simulink model "ev_tms_v4"  (R2023a)
settings: Solver=VariableStepAuto  StartTime=0.0  StopTime=inf  RelTol=1e-3  AbsTol=1e-3
model workspace: external: MATLAB File /Users/rossschrader/Desktop/ML/ME/_Project/_v3/ev_tms_v3_params.m (data not in the file)
values from neighbouring files (symbols this model uses):
  ac_onoff = 0    [ev_tms_v4_params.m]
  battery_C1_LUT = [ ... (first row only)    [ev_tms_v4_params.m]
  battery_capacity_LUT = [28.0081 27.6250 27.6392]    [ev_tms_v4_params.m]
  battery_cell_cp = 795    [ev_tms_v4_params.m]
  battery_cell_mass = 2.5    [ev_tms_v4_params.m]
  battery_Em_LUT = [ ... (first row only)    [ev_tms_v4_params.m]
  battery_N_cells = 20    [ev_tms_v4_params.m]
  battery_Qe_init = 0    [ev_tms_v4_params.m]
  battery_R0_LUT = [ ... (first row only)    [ev_tms_v4_params.m]
  battery_R1_LUT = [ ... (first row only)    [ev_tms_v4_params.m]
  battery_SOC_LUT = [0 0.1 0.25 0.5 0.75 0.9 1]'    [ev_tms_v4_params.m]
  battery_T_init = init_T    (= 21)    [ev_tms_v4_params.m]
  battery_temperature_LUT = [5 20 40]    [ev_tms_v4_params.m]
  cabin_duct_area = 0.04    [ev_tms_v4_params.m]
  cabin_T_init = init_T    (= 21)    [ev_tms_v4_params.m]
  chiller_area_primary = chiller_N_tubes * pi * chiller_tube_D * chiller_tube_L    (= 0.439822971503)    [ev_tms_v4_params.m]
  chiller_N_baffles = 3    [ev_tms_v4_params.m]
  chiller_N_tubes = 100    [ev_tms_v4_params.m]
  chiller_tube_D = 0.0035    [ev_tms_v4_params.m]
  chiller_tube_L = 0.4    [ev_tms_v4_params.m]
  chiller_wall_conductivity = 240    [ev_tms_v4_params.m]
  chiller_wall_thickness = 1e-4    (= 0.0001)    [ev_tms_v4_params.m]
  compressor_rpm_LUT = [0, 1800, 3600]    [ev_tms_v4_params.m]
  condenser_air_area_flow = (condenser_N_tubes - 1) * condenser_L * condenser_gap_H    (= 0.3906)    [ev_tms_v4_params.m]
  condenser_air_area_primary = 2 * (condenser_N_tubes - 1) * condenser_W * (condenser_L + condenser_gap_H)    (= 1.4835)    [ev_tms_v4_params.m]
  condenser_W = 0.015    [ev_tms_v4_params.m]
  condenser_wall_conductivity = 240    [ev_tms_v4_params.m]
  condenser_wall_thickness = 1e-4    (= 0.0001)    [ev_tms_v4_params.m]
  coolant_channel_D = 0.0092    [ev_tms_v4_params.m]
  coolant_pipe_D = 0.019    [ev_tms_v4_params.m]
  coolant_T_init = init_T    (= 21)    [ev_tms_v4_params.m]
  coolant_tank_area = 0.11^2    (= 0.0121)    [ev_tms_v4_params.m]
  coolant_tank_volume = 5    [ev_tms_v4_params.m]
  coolant_valve_D_ratio_max = 0.95    [ev_tms_v4_params.m]
  coolant_valve_D_ratio_min = 1e-3    (= 0.001)    [ev_tms_v4_params.m]
  coolant_valve_displacement = 0.0063    [ev_tms_v4_params.m]
  coolant_valve_S_max = 0.0053    [ev_tms_v4_params.m]
  evaporator_air_area_flow = (evaporator_N_tubes - 1) * evaporator_L * evaporator_gap_H    (= 0.12)    [ev_tms_v4_params.m]
  evaporator_air_area_primary = 2 * (evaporator_N_tubes - 1) * evaporator_W * (evaporator_L + evaporator_gap_H)    (= 0.4323)    [ev_tms_v4_params.m]
  evaporator_P_target = 0.3    [ev_tms_v4_params.m]
  evaporator_W = 0.015    [ev_tms_v4_params.m]
  evaporator_wall_conductivity = 240    [ev_tms_v4_params.m]
  evaporator_wall_thickness = 1e-4    (= 0.0001)    [ev_tms_v4_params.m]
  pump_speed_max = 1000    [ev_tms_v4_params.m]
  radiator_air_area_flow = (radiator_N_tubes - 1) * radiator_L * radiator_gap_H    (= 0.0975)    [ev_tms_v4_params.m]
  radiator_air_area_primary = 2 * (radiator_N_tubes - 1) * radiator_W * (radiator_L + radiator_gap_H)    (= 0.436875)    [ev_tms_v4_params.m]
  radiator_W = 0.015    [ev_tms_v4_params.m]
  radiator_wall_conductivity = 240    [ev_tms_v4_params.m]
  radiator_wall_thickness = 1e-4    (= 0.0001)    [ev_tms_v4_params.m]
  refrigerant_alpha_init = 0.6    [ev_tms_v4_params.m]
  refrigerant_pipe_D = 0.01    [ev_tms_v4_params.m]
  T_env = t_(x)    [ev_tms_v4_params.m]
  T_setpoint = 20    [ev_tms_v4_params.m]
undefined symbols (not defined in the file or in its folder): bulb, outlet
libraries: fl_lib x221, nesl_utility x79, SimscapeFluids_lib x25, LiBatteryElements_lib x16, sdl_lib x3, slpidlib x2, simulink x1, rllib x1, autolibshared x1, SignalEditorBlockLib x1
(part 2 of 8)

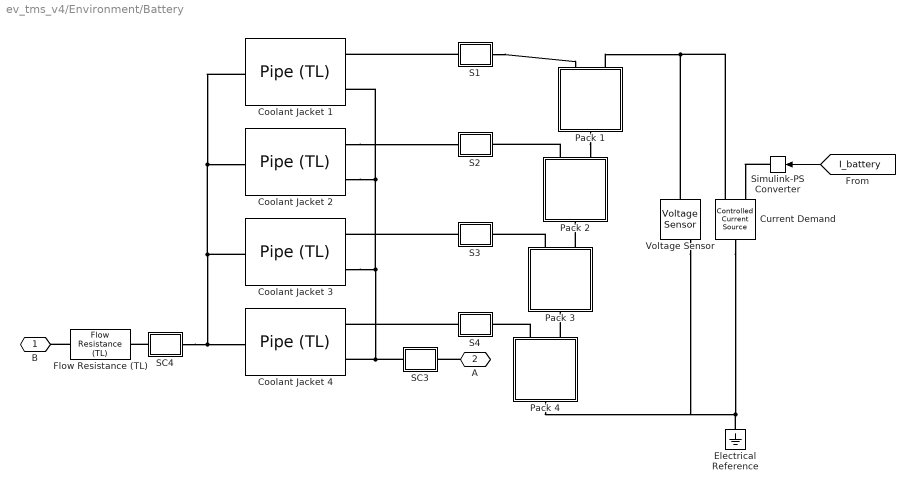
== system ev_tms_v4/Environment/Battery ==
  Coolant Jacket {1..4} (4 alike) : SimscapeFluids_lib/Thermal Liquid/Pipes & Fittings/Pipe (TL)  dynamic_compressibility=simscape.enum.onoff.on  inertia=simscape.enum.onoff.off  num_segments=1  pipe_length=0.7 m  cross_section_geometry=fluids.thermal_liquid.pipes_fittings.enum.CrossSectionGeometry.Custom  pipe_diameter=0.1 m  pipe_inner_diameter=0.05 m  pipe_outer_diameter=0.1 m  pipe_width=0.1 m  pipe_height=0.1 m  pipe_major_axis=0.1 m  pipe_minor_axis=0.05 m  pipe_side=0.1 m  pipe_angle=30 deg  area=pi * coolant_channel_D^2 / 4 m^2  Dh=coolant_channel_D m  wall_spec=fluids.thermal_liquid.pipes_fittings.enum.wall_spec.rigid  wall_compliance=1.2e-6 m/MPa  wall_time_constant=0.01 s  elevation_spec=foundation.enum.constant_variable.constant  elevation_gain=0 m  g=9.81 m/s^2  pressure_loss_spec=fluids.thermal_liquid.pipes_fittings.enum.PressureLossSpec.Haaland  local_pressure_loss_spec=fluids.thermal_liquid.pipes_fittings.enum.LocalLossSpec.AggregateLength  length_add=0 m  loss_coefficient=0.1  roughness_spec=fluids.thermal_liquid.pipes_fittings.enum.RoughnessSpec.Custom  roughness=1.5e-5 m  Re_friction_TLU=[ 400 1000 1.5e+3 3e+3 4e+3 6e+3 1e+4 2e+4 4e+4 6e+4 1e+5 1e+8 ]  friction_factor_TLU=[ 0.264 0.112 0.07099999999999999 0.0417 0.0387 0.0268 0.025 0.0232 0.0226 0.022 0.0214 0.0214 ]  shape_factor=64  Re_lam=100  Re_tur=500  mdot_nominal=[ 0.1 1 ] kg/s  p_diff_nominal=[ 0.001 0.01 ] MPa  mdot_threshold=1e-6 kg/s  heat_transfer_spec=fluids.thermal_liquid.pipes_fittings.enum.HeatTransferSpec.DittusBoelter  mdot_nominal_heat=[ 0.1 1 ] kg/s  T_in_nominal=[ 293.15 293.15 ] K  T_out_nominal=[ 300 300 ] K  p_in_nominal_heat=[ 0.101325 0.101325 ] MPa  T_wall_nominal=[ 303.15 303.15 ] K  a_coeff=0.3  b_Re_power=0.8  c_Pr_power=0.33  Nu_lam=3.66  Re_Colburn_TLU=[ 100 150 1000 ]  Colburn_factor_TLU=[ 0.019 0.013 0.002 ]  Re_Nu_TLU=[ 100 150 1000 ]  Pr_Nu_TLU=[ 1 10 ]  Nu_TLU=[ 3.72 4.21; 3.75 4.44; 4.21 7.15 ]  p0_vec=coolant_p_init MPa  T0_vec=coolant_T_init degC  mdot0=0.1 kg/s
  Current Demand : fl_lib/Electrical/Electrical Sources/Controlled Current Source
  Electrical Reference : fl_lib/Electrical/Electrical Elements/Electrical Reference
  Flow Resistance (TL) : fl_lib/Thermal Liquid/Elements/Flow Resistance (TL)  delta_p_nominal=1e-5 MPa  mdot_nominal=0.02 kg/s  area=pi * coolant_pipe_D^2 / 4 m^2  laminar_fraction=1e-3
  Pack 1 : Subsystem  Tag=PublishSubsystem  mask(Lithium cell (one RC-branch equivalent circuit)){Ncells=battery_N_cells, Qe_init=battery_Qe_init, T_init=battery_T_init + 273.15, Capacity_LUT=battery_capacity_LUT, Em_LUT=battery_Em_LUT, R0_LUT=battery_R0_LUT, R1_LUT=battery_R1_LUT, C1_LUT=battery_C1_LUT, cell_mass=battery_cell_mass, cell_Cp_heat=battery_cell_cp, SOC_LUT=battery_SOC_LUT, Temperature_LUT=battery_temperature_LUT + 273.15}
      mask prompts: Ncells "Number of series-connected cells"; Qe_init "Initial cell charge deficit (A*hr)"; T_init "Initial cell temperature (K)"; Capacity_LUT "Capacity (A*hr, 1xN table)"; Em_LUT "Em open-circuit voltage, Em (volts, MxN table)"; R0_LUT "R0 terminal resistance (ohms, MxN table)"; R1_LUT "R1 cell resistance (ohms, MxN table)"; C1_LUT "C1 capacitance (farads, MxN table)"; cell_mass "Cell mass (kg)"; cell_Cp_heat "Cell specific heat (J/kg/K)"; SOC_LUT "SOC table breakpoints (Mx1 array)"; Temperature_LUT "Temperature table breakpoints (K, 1xN array)"
      mask DialogControl ParameterTabVar0 Prompt: Main
      mask DialogControl ParameterTabVar01 Prompt: Electrical (per cell)
      mask DialogControl ParameterTabVar012 Prompt: Thermal (per cell)
      mask DialogControl ParameterTabVar0123 Prompt: Table Breakpoints
      mask Display:
      | % Battery icon
      | plot([2.8 1.3], [0 0])
      | plot([-0.2 -1.2 -1.2 -2.8], [0 0 -0.8 -0.8])
      | patch([1 1 -1 -1]*0.15 + 1.6, [-1 1 1 -1]*0.4, [0 0 0])
      | patch([1 1 -1 -1]*0.15 + 0.4, [-1 1 1 -1]*0.4, [0 0 0])
      | patch([1 1 -1 -1]*0.15 + 1.0, [-1 1 1 -1]*0.8, [0 0 0])
      | patch([1 1 -1 -1]*0.15 - 0.2, [-1 1 1 -1]*0.8, [0 0 0])
      | 
      | % Thermal port
      | plot([-1.4 -0.8], [1.2 1.2])
      | plot([-1.4 -0.8], [0.5 0.5])
      | plot([-1.4 -2.8], [0.8 0.8])
      | plot(0.2*sin(0:2*pi/50:2*pi) - 1.4, 0.35*cos(0:2*pi/50:2*pi) + 0.85)
      | plot(0.2*sin(0:2*pi/50:pi) - 0.8, 0.35*cos(0:2*pi/50:pi) + 0.85)
      | 
      | % Plot points to set plot range
      | color('white')
      | plot(2.8, 1.6)
      | plot(-2.8, -1.6)
      | 
      | % Port labels
      | color('red')
      | port_label('LConn', 1, 'H')
      | port_label('LConn', 2, '+')
      | port_label('RConn', 1, '-')
  Pack 2 : Subsystem  mask(Lithium cell (one RC-branch equivalent circuit)){Ncells=battery_N_cells, Qe_init=battery_Qe_init, T_init=battery_T_init + 273.15, Capacity_LUT=battery_capacity_LUT, Em_LUT=battery_Em_LUT, R0_LUT=battery_R0_LUT, R1_LUT=battery_R1_LUT, C1_LUT=battery_C1_LUT, cell_mass=battery_cell_mass, cell_Cp_heat=battery_cell_cp, SOC_LUT=battery_SOC_LUT, Temperature_LUT=battery_temperature_LUT + 273.15}
      mask prompts: Ncells "Number of series-connected cells"; Qe_init "Initial cell charge deficit (A*hr)"; T_init "Initial cell temperature (K)"; Capacity_LUT "Capacity (A*hr, 1xN table)"; Em_LUT "Em open-circuit voltage, Em (volts, MxN table)"; R0_LUT "R0 terminal resistance (ohms, MxN table)"; R1_LUT "R1 cell resistance (ohms, MxN table)"; C1_LUT "C1 capacitance (farads, MxN table)"; cell_mass "Cell mass (kg)"; cell_Cp_heat "Cell specific heat (J/kg/K)"; SOC_LUT "SOC table breakpoints (Mx1 array)"; Temperature_LUT "Temperature table breakpoints (K, 1xN array)"
      mask DialogControl ParameterTabVar0 Prompt: Main
      mask DialogControl ParameterTabVar01 Prompt: Electrical (per cell)
      mask DialogControl ParameterTabVar012 Prompt: Thermal (per cell)
      mask DialogControl ParameterTabVar0123 Prompt: Table Breakpoints
      mask Display:
      | % Battery icon
      | plot([2.8 1.3], [0 0])
      | plot([-0.2 -1.2 -1.2 -2.8], [0 0 -0.8 -0.8])
      | patch([1 1 -1 -1]*0.15 + 1.6, [-1 1 1 -1]*0.4, [0 0 0])
      | patch([1 1 -1 -1]*0.15 + 0.4, [-1 1 1 -1]*0.4, [0 0 0])
      | patch([1 1 -1 -1]*0.15 + 1.0, [-1 1 1 -1]*0.8, [0 0 0])
      | patch([1 1 -1 -1]*0.15 - 0.2, [-1 1 1 -1]*0.8, [0 0 0])
      | 
      | % Thermal port
      | plot([-1.4 -0.8], [1.2 1.2])
      | plot([-1.4 -0.8], [0.5 0.5])
      | plot([-1.4 -2.8], [0.8 0.8])
      | plot(0.2*sin(0:2*pi/50:2*pi) - 1.4, 0.35*cos(0:2*pi/50:2*pi) + 0.85)
      | plot(0.2*sin(0:2*pi/50:pi) - 0.8, 0.35*cos(0:2*pi/50:pi) + 0.85)
      | 
      | % Plot points to set plot range
      | color('white')
      | plot(2.8, 1.6)
      | plot(-2.8, -1.6)
      | 
      | % Port labels
      | color('red')
      | port_label('LConn', 1, 'H')
      | port_label('LConn', 2, '+')
      | port_label('RConn', 1, '-')
  Pack 3 : Subsystem  mask(Lithium cell (one RC-branch equivalent circuit)){Ncells=battery_N_cells, Qe_init=battery_Qe_init, T_init=battery_T_init + 273.15, Capacity_LUT=battery_capacity_LUT, Em_LUT=battery_Em_LUT, R0_LUT=battery_R0_LUT, R1_LUT=battery_R1_LUT, C1_LUT=battery_C1_LUT, cell_mass=battery_cell_mass, cell_Cp_heat=battery_cell_cp, SOC_LUT=battery_SOC_LUT, Temperature_LUT=battery_temperature_LUT + 273.15}
      mask prompts: Ncells "Number of series-connected cells"; Qe_init "Initial cell charge deficit (A*hr)"; T_init "Initial cell temperature (K)"; Capacity_LUT "Capacity (A*hr, 1xN table)"; Em_LUT "Em open-circuit voltage, Em (volts, MxN table)"; R0_LUT "R0 terminal resistance (ohms, MxN table)"; R1_LUT "R1 cell resistance (ohms, MxN table)"; C1_LUT "C1 capacitance (farads, MxN table)"; cell_mass "Cell mass (kg)"; cell_Cp_heat "Cell specific heat (J/kg/K)"; SOC_LUT "SOC table breakpoints (Mx1 array)"; Temperature_LUT "Temperature table breakpoints (K, 1xN array)"
      mask DialogControl ParameterTabVar0 Prompt: Main
      mask DialogControl ParameterTabVar01 Prompt: Electrical (per cell)
      mask DialogControl ParameterTabVar012 Prompt: Thermal (per cell)
      mask DialogControl ParameterTabVar0123 Prompt: Table Breakpoints
      mask Display:
      | % Battery icon
      | plot([2.8 1.3], [0 0])
      | plot([-0.2 -1.2 -1.2 -2.8], [0 0 -0.8 -0.8])
      | patch([1 1 -1 -1]*0.15 + 1.6, [-1 1 1 -1]*0.4, [0 0 0])
      | patch([1 1 -1 -1]*0.15 + 0.4, [-1 1 1 -1]*0.4, [0 0 0])
      | patch([1 1 -1 -1]*0.15 + 1.0, [-1 1 1 -1]*0.8, [0 0 0])
      | patch([1 1 -1 -1]*0.15 - 0.2, [-1 1 1 -1]*0.8, [0 0 0])
      | 
      | % Thermal port
      | plot([-1.4 -0.8], [1.2 1.2])
      | plot([-1.4 -0.8], [0.5 0.5])
      | plot([-1.4 -2.8], [0.8 0.8])
      | plot(0.2*sin(0:2*pi/50:2*pi) - 1.4, 0.35*cos(0:2*pi/50:2*pi) + 0.85)
      | plot(0.2*sin(0:2*pi/50:pi) - 0.8, 0.35*cos(0:2*pi/50:pi) + 0.85)
      | 
      | % Plot points to set plot range
      | color('white')
      | plot(2.8, 1.6)
      | plot(-2.8, -1.6)
      | 
      | % Port labels
      | color('red')
      | port_label('LConn', 1, 'H')
      | port_label('LConn', 2, '+')
      | port_label('RConn', 1, '-')
  Pack 4 : Subsystem  mask(Lithium cell (one RC-branch equivalent circuit)){Ncells=battery_N_cells, Qe_init=battery_Qe_init, T_init=battery_T_init + 273.15, Capacity_LUT=battery_capacity_LUT, Em_LUT=battery_Em_LUT, R0_LUT=battery_R0_LUT, R1_LUT=battery_R1_LUT, C1_LUT=battery_C1_LUT, cell_mass=battery_cell_mass, cell_Cp_heat=battery_cell_cp, SOC_LUT=battery_SOC_LUT, Temperature_LUT=battery_temperature_LUT + 273.15}
      mask prompts: Ncells "Number of series-connected cells"; Qe_init "Initial cell charge deficit (A*hr)"; T_init "Initial cell temperature (K)"; Capacity_LUT "Capacity (A*hr, 1xN table)"; Em_LUT "Em open-circuit voltage, Em (volts, MxN table)"; R0_LUT "R0 terminal resistance (ohms, MxN table)"; R1_LUT "R1 cell resistance (ohms, MxN table)"; C1_LUT "C1 capacitance (farads, MxN table)"; cell_mass "Cell mass (kg)"; cell_Cp_heat "Cell specific heat (J/kg/K)"; SOC_LUT "SOC table breakpoints (Mx1 array)"; Temperature_LUT "Temperature table breakpoints (K, 1xN array)"
      mask DialogControl ParameterTabVar0 Prompt: Main
      mask DialogControl ParameterTabVar01 Prompt: Electrical (per cell)
      mask DialogControl ParameterTabVar012 Prompt: Thermal (per cell)
      mask DialogControl ParameterTabVar0123 Prompt: Table Breakpoints
      mask Display:
      | % Battery icon
      | plot([2.8 1.3], [0 0])
      | plot([-0.2 -1.2 -1.2 -2.8], [0 0 -0.8 -0.8])
      | patch([1 1 -1 -1]*0.15 + 1.6, [-1 1 1 -1]*0.4, [0 0 0])
      | patch([1 1 -1 -1]*0.15 + 0.4, [-1 1 1 -1]*0.4, [0 0 0])
      | patch([1 1 -1 -1]*0.15 + 1.0, [-1 1 1 -1]*0.8, [0 0 0])
      | patch([1 1 -1 -1]*0.15 - 0.2, [-1 1 1 -1]*0.8, [0 0 0])
      | 
      | % Thermal port
      | plot([-1.4 -0.8], [1.2 1.2])
      | plot([-1.4 -0.8], [0.5 0.5])
      | plot([-1.4 -2.8], [0.8 0.8])
      | plot(0.2*sin(0:2*pi/50:2*pi) - 1.4, 0.35*cos(0:2*pi/50:2*pi) + 0.85)
      | plot(0.2*sin(0:2*pi/50:pi) - 0.8, 0.35*cos(0:2*pi/50:pi) + 0.85)
      | 
      | % Plot points to set plot range
      | color('white')
      | plot(2.8, 1.6)
      | plot(-2.8, -1.6)
      | 
      | % Port labels
      | color('red')
      | port_label('LConn', 1, 'H')
      | port_label('LConn', 2, '+')
      | port_label('RConn', 1, '-')
  S1 : Subsystem
      mask Display: disp(get_param(gcb, 'Name'))
  S2 : Subsystem
      mask Display: disp(get_param(gcb, 'Name'))
  S3 : Subsystem
      mask Display: disp(get_param(gcb, 'Name'))
  S4 : Subsystem
      mask Display: disp(get_param(gcb, 'Name'))
  SC3 : Subsystem
      mask Display: disp(get_param(gcb, 'Name'))
  SC4 : Subsystem
      mask Display: disp(get_param(gcb, 'Name'))
  Simulink-PS Converter : nesl_utility/Simulink-PS Converter  PhysicalDomain=network_engine_domain  SubClassName=ps_input  LeftPortType=input  RightPortType=output  PseudoPeriodic=off  Frequencies=[]  NoiseDistribution=none  NoiseParameters=[]  Unit=A  AffineConversion=off  FilteringAndDerivatives=provide  SimscapeFilterOrder=1  InputFilterTimeConstant=0.001  UdotUserProvided=0
  Voltage Sensor : fl_lib/Electrical/Electrical Sensors/Voltage Sensor
  B : PMIOPort  Side=Left
  A : PMIOPort  Port=2  Side=Right
  wires:
  [I_battery] -> Simulink-PS Converter/1
  connections:
  Current Demand/LConn1 -- Pack 4/RConn1 -- Voltage Sensor/RConn2 -- Electrical Reference/LConn1
  Current Demand/RConn2 -- Pack 1/LConn2 -- Voltage Sensor/LConn1
  Simulink-PS Converter/RConn1 -- Current Demand/RConn1
  S1/LConn1 -- Coolant Jacket 1/LConn2
  S3/LConn1 -- Coolant Jacket 3/LConn2
  S4/LConn1 -- Coolant Jacket 4/LConn2
  Pack 1/RConn1 -- Pack 2/LConn2
  Pack 3/LConn2 -- Pack 2/RConn1
  Pack 4/LConn2 -- Pack 3/RConn1
  Pack 2/LConn1 -- S2/RConn1
  Coolant Jacket 3/LConn1 -- SC3/LConn1 -- Coolant Jacket 4/LConn1 -- Coolant Jacket 1/LConn1 -- Coolant Jacket 2/LConn1
  S1/RConn1 -- Pack 1/LConn1
  Coolant Jacket 2/LConn2 -- S2/LConn1
  Pack 3/LConn1 -- S3/RConn1
  Pack 4/LConn1 -- S4/RConn1
  A/RConn1 -- SC3/RConn1
  Coolant Jacket 3/RConn1 -- Coolant Jacket 2/RConn1 -- Coolant Jacket 1/RConn1 -- SC4/RConn1 -- Coolant Jacket 4/RConn1
  SC4/LConn1 -- Flow Resistance (TL)/LConn1
  Flow Resistance (TL)/RConn1 -- B/RConn1

== system ev_tms_v4/Environment/Battery Pump ==
  Battery Pump : SimscapeFluids_lib/Thermal Liquid/Pumps & Motors/Fixed-Displacement Pump (TL)  loss_spec=1  displacement=pump_displacement l/rev  omega_nominal=0.5 * pump_speed_max rpm  p_nominal=0.1 MPa  mu_nominal=0.9 cP  vol_eff_nominal=0.92  mech_eff_nominal=0.88  no_load_torque=0.03 N*m  p_diff_eff_TLU=[.1, 1, 2] MPa  omega_eff_TLU=[25, 50, 100, 200, 300, 400] rad/s  vol_eff_TLU=[.816, .908, .954, .977, .981, .984; .325, .663, .831, .916, .925, .946; .137, .568, .78, .892, .893, .91]  mech_eff_TLU=[.996, .996, .996, .996, .996, .996; .988, .989, .989, .989, .989, .99; .981, .981, .982, .982, .983, .984]  p_diff_loss_TLU=[.1, 1, 2] MPa  omega_loss_TLU=[25, 50, 100, 200, 300, 400] rad/s  vol_loss_TLU=[.023, .023, .023, .023, .0285, .032; .0844, .0842, .0845, .084, .1125, .108; .1079, .108, .11, .108, .1605, .18] * 1e-3 m^3/s  mech_loss_TLU=[.002, .002, .002, .002, .002, .002; .0607, .0556, .0556, .0556, .0556, .0505; .1937, .1937, .1833, .1833, .1729, .1626] N*m  vol_eff_min=1e-3  vol_eff_max=1  mech_eff_min=1e-3  mech_eff_max=1  pressure_threshold=1e-3 MPa  omega_threshold=10 rad/s  area=pi * coolant_pipe_D^2 / 4 m^2  quadrant_check=0  pump_mode_check=simscape.enum.assert.action.none
  From1 : From  Commented=on  GotoTag=cmd_battery_pump_2
  Ideal Angular Velocity Source : fl_lib/Mechanical/Mechanical Sources/Ideal Angular Velocity Source
  Max Speed [rpm] : Gain  Gain=pump_speed_max
  Mechanical Rotational Reference : fl_lib/Mechanical/Rotational Elements/Mechanical Rotational Reference
  PS-Simulink Converter : nesl_utility/PS-Simulink Converter  PhysicalDomain=network_engine_domain  SubClassName=ps_output  LeftPortType=input  RightPortType=output  PseudoPeriodic=off  Frequencies=[]  VectorFormat=inherit  Unit=inherit  AffineConversion=off
  Rotational Power Sensor : sdl_lib/Sensors/Rotational Power Sensor  measurement_type=sdl.enum.rotationalPowerSensorType.instantaneous  averaging_period=1 s  max_frequency=1000 Hz  max_speed=1000 rpm
      settings: InternalSimscapePortConfiguration="{\"Bottom\":[],\"Left\":[{\"id\":\"S\",\"label\":\"S\",\"type\":\"foundation.mechanical.rotational.rotational\"},{\"id\":\"R\",\"label\":\"R\",\"type\":\"foundation.mechanical.rotational.rotational\"},{\"id\":\"C\",\"label\":\"C\",\"type\":\"foundation.mechanical.rotational.rotational\"}],\"Right\":[{\"id\":\"P\",\"label\":\"P\",\"type\":\"output\"}],\"Top\":[]}"
  Simulink-PS Converter : nesl_utility/Simulink-PS Converter  PhysicalDomain=network_engine_domain  SubClassName=ps_input  LeftPortType=input  RightPortType=output  PseudoPeriodic=off  Frequencies=[]  NoiseDistribution=none  NoiseParameters=[]  Unit=rpm  AffineConversion=off  FilteringAndDerivatives=provide  SimscapeFilterOrder=1  InputFilterTimeConstant=0.001  UdotUserProvided=0
  Transfer Fcn : TransferFcn  Denominator=[5 1]
  A : PMIOPort  Side=Left
  B : PMIOPort  Port=2  Side=Right
  tag scope: bat_pump_pwr=global
  wires:
  Max Speed [rpm]/1 -> Simulink-PS Converter/1
  Transfer Fcn/1 -> Max Speed [rpm]/1
  PS-Simulink Converter/1 -> [bat_pump_pwr]
  [cmd_battery_pump] -> Transfer Fcn/1
  connections:
  Battery Pump/LConn2 -- B/RConn1
  Battery Pump/LConn1 -- A/RConn1
  Battery Pump/RConn2 -- Rotational Power Sensor/LConn3 -- Mechanical Rotational Reference/LConn1 -- Ideal Angular Velocity Source/RConn2
  Simulink-PS Converter/RConn1 -- Ideal Angular Velocity Source/RConn1
  Ideal Angular Velocity Source/LConn1 -- Rotational Power Sensor/LConn1
  Battery Pump/RConn1 -- Rotational Power Sensor/LConn2
  PS-Simulink Converter/LConn1 -- Rotational Power Sensor/RConn1

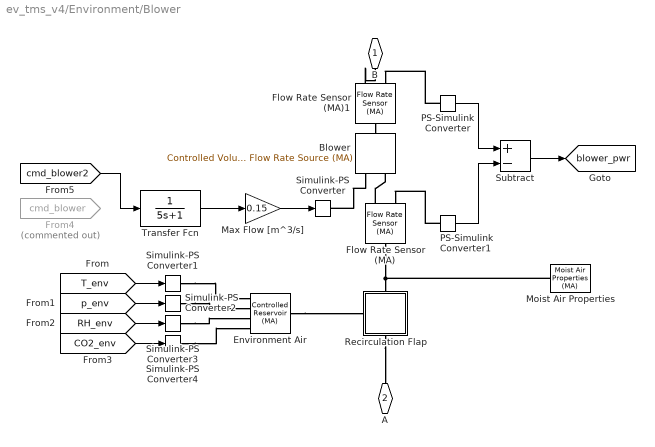
== system ev_tms_v4/Environment/Blower ==
  Blower : fl_lib/Moist Air/Sources/Controlled Volumetric Flow Rate Source (MA)  power_spec=foundation.enum.power_spec.isentropic  volumetric_flow_conditions=foundation.enum.volumetric_flow_conditions.actual  p_std=0.101325 MPa  T_std=20 degC  RH_std=0.65  area_A=cabin_duct_area m^2  area_B=cabin_duct_area m^2
      settings: InternalSimscapePortConfiguration="{\"Bottom\":[],\"Left\":[{\"id\":\"A\",\"label\":\"A\",\"type\":\"foundation.moist_air.moist_air\"},{\"id\":\"V\",\"label\":\"V\",\"type\":\"input\"}],\"Right\":[{\"id\":\"B\",\"label\":\"B\",\"type\":\"foundation.moist_air.moist_air\"}],\"Top\":[]}"
  Environment Air : fl_lib/Moist Air/Elements/Controlled Reservoir (MA)  moisture_spec=foundation.enum.moisture_spec.relative_humidity  trace_gas_spec=foundation.enum.trace_gas_spec.mole_fraction  RH_ws=1  area_A=cabin_duct_area m^2  input_error_spec=foundation.enum.input_range_error.warn
      settings: InternalSimscapePortConfiguration="{\"Bottom\":[],\"Left\":[{\"id\":\"A\",\"label\":\"A\",\"type\":\"foundation.moist_air.moist_air\"}],\"Right\":[{\"id\":\"T\",\"label\":\"T\",\"type\":\"input\"},{\"id\":\"P\",\"label\":\"P\",\"type\":\"input\"},{\"id\":\"W\",\"label\":\"W\",\"type\":\"input\"},{\"id\":\"G\",\"label\":\"G\",\"type\":\"input\"}],\"Top\":[]}"
  Flow Rate Sensor (MA) : fl_lib/Moist Air/Sensors/Flow Rate Sensor (MA)  mass_flow_measure=false  volumetric_flow_measure=false  volumetric_flow_conditions=foundation.enum.volumetric_flow_conditions.actual  p_std=0.101325 MPa  T_std=20 degC  RH_std=0.65  energy_flow_measure=true  vapor_flow_measure=false  gas_flow_measure=false
      settings: InternalSimscapePortConfiguration="{\"Bottom\":[{\"id\":\"PHI\",\"label\":\"φ\",\"type\":\"output\"}],\"Left\":[{\"id\":\"A\",\"label\":\"A\",\"type\":\"foundation.moist_air.moist_air\"}],\"Right\":[{\"id\":\"B\",\"label\":\"B\",\"type\":\"foundation.moist_air.moist_air\"}],\"Top\":[]}"
  Flow Rate Sensor (MA)1 : fl_lib/Moist Air/Sensors/Flow Rate Sensor (MA)  mass_flow_measure=false  volumetric_flow_measure=false  volumetric_flow_conditions=foundation.enum.volumetric_flow_conditions.actual  p_std=0.101325 MPa  T_std=20 degC  RH_std=0.65  energy_flow_measure=true  vapor_flow_measure=false  gas_flow_measure=false
      settings: InternalSimscapePortConfiguration="{\"Bottom\":[{\"id\":\"PHI\",\"label\":\"φ\",\"type\":\"output\"}],\"Left\":[{\"id\":\"A\",\"label\":\"A\",\"type\":\"foundation.moist_air.moist_air\"}],\"Right\":[{\"id\":\"B\",\"label\":\"B\",\"type\":\"foundation.moist_air.moist_air\"}],\"Top\":[]}"
  From4 : From  Commented=on  GotoTag=cmd_blower  TagVisibility=global
  Max Flow [m^3/s] : Gain  Gain=0.15
  Moist Air Properties : fl_lib/Moist Air/Utilities/Moist Air Properties (MA)  R_a=287.047 J/kg/K  T_TLU=[-56.55, -50 : 10 : -10, -5 : 1 : 5, 10 : 10 : 350]' degC  h_a_TLU=[342.416126230579; 349.005511058471; 359.063577249119; 369.119948684177; 379.175469465129; 389.230944678417; 394.258910928084; 395.264534937366; 396.27017101329; 397.275819932805; 398.281482472874; 399.287159410541; 400.292851523015; 401.298559587728; 402.304284382408; 403.310026685143; 404.315787274435; 409.34489180313; 419.404921755863; 429.468036401264; 439.535033154839; 449.606720928652; 459.683919949603; 469.767460521911; 479.858181001348; 489.956925196484; 500.064539372946; 510.181869006204; 520.309755403634; 530.449032296018; 540.60052248087; 550.765034584465; 560.943359995745; 571.136270013102; 581.344513234296; 591.568813210327; 601.809866375885; 612.068340261954; 622.344871990218; 632.640067043998; 642.95449830646; 653.288705353699; 663.643193987949; 674.018435994423; 684.414869104228; 694.832897145098; 705.272890361557; 715.735185886199; 726.220088344236; 736.727870574087; 747.258774447567; 757.813011774199] kJ/kg  mu_a_TLU=[14.2568883320012; 14.6140127728333; 15.1517277055779; 15.6806860159119; 16.2012351072083; 16.7137043125028; 16.9670071730589; 17.017438062815; 17.0677930842452; 17.1180725309876; 17.1682766951315; 17.2184058672268; 17.2684603362935; 17.3184403898301; 17.3683463138234; 17.4181783927569; 17.4679369096204; 17.7156358640698; 18.2056751785154; 18.68879035749; 19.1652344664982; 19.6352478927873; 20.099059103658; 20.5568853601578; 21.0089333871663; 21.4554000014051; 21.8964726992323; 22.3323302062775; 22.7631429910631; 23.1890737447833; 23.6102778293792; 24.0269036959922; 24.4390932757886; 24.8469823450548; 25.2507008663546; 25.6503733074314; 26.0461189394339; 26.4380521159325; 26.8262825340948; 27.2109154792923; 27.5920520543128; 27.969789394274; 28.3442208682439; 28.7154362685068; 29.0835219883356; 29.4485611890712; 29.8106339572472; 30.1698174524429; 30.5261860464955; 30.8798114546565; 31.2307628592324; 31.5791070262086] s*uPa  k_a_TLU=[19.8808489374933; 20.4162454629695; 21.2248743590758; 22.0232452890903; 22.8117314495857; 23.5906913619588; 23.9767075412237; 24.053639990175; 24.1304826682191; 24.2072359051629; 24.2839000294007; 24.3604753679152; 24.4369622462801; 24.5133609886625; 24.5896719178249; 24.6658953551279; 24.7420316205333; 25.1214164701832; 25.8738283029331; 26.6180150229276; 27.3542674377332; 28.0828634735341; 28.8040686837224; 29.5181367785657; 30.2253101618423; 30.9258204644224; 31.6198890677835; 32.3077276126633; 32.9895384896798; 33.6655153099498; 34.33584335461; 35.0007000027879; 35.6602551380254; 36.3146715334901; 36.9641052165342; 37.6087058133173; 38.248616874307; 38.8839761815308; 39.5149160384798; 40.1415635435708; 40.7640408480637; 41.3824653993118; 41.9969501701893; 42.6076038755117; 43.2145311762238; 43.8178328720941; 44.4176060836121; 45.013944423749; 45.6069381602018; 46.1966743687041; 46.783237077953; 47.3667074066625] mW/m/K  p_min=1 kPa  p_max=inf MPa  T_min=-56.55 degC  T_max=350 degC  properties_range_check=simscape.enum.assert.action.error  p_atm=0.101325 MPa  T_atm=20 degC  R_w=461.523 J/kg/K  p_ws_TLU=[1.71168953425982e-06; 3.93770601979424e-06; 1.28411717710344e-05; 3.80051394873809e-05; .00010323902900209; .000259873810798063; .000401741022116384; .000437454836117844; .000476040820618202; .000517704666185737; .000562664883741207; .000611212677444345; .000657088049117899; .000705987905898279; .000758082381149132; .000813549384183233; .000872574861129522; .00122818386934022; .0023392147667769; .00424668834054807; .00738442748706953; .0123512704340234; .0199458019246787; .0312006356960619; .0474147199263783; .0701823607447713; .10141797792131; .143375967241115; .198665399739302; .270259606559999; .361500961984849; .476101381081492; .618139196722055; .792053183687694; 1.0026345688121; 1.25501792086105; 1.55467186826983; 1.90739066433297; 2.31928772772542; 2.79679245576864; 3.34665187151016; 3.97593907083533; 4.69207105435535; 5.5028394740883; 6.41645928168037; 7.4416425436169; 8.58770832955728; 9.86474556030261; 11.2838558865497; 12.8575218898034; 14.6001810568052; 16.5291642526045] MPa  h_w_vap_TLU=[2836.88241275372; 2837.81392500514; 2838.63937175807; 2838.7309929628; 2838.06905313927; 2836.62597341095; 2835.60023952573; 2835.37006381376; 2835.13143158077; 2834.88429145066; 2834.62859062897; 2500.93420564316; 2498.55329907119; 2496.17495082036; 2493.79885912205; 2491.42474723191; 2489.05236104642; 2477.20875029194; 2453.54955988604; 2429.83856603313; 2406.00136954922; 2381.97406342174; 2357.69101156389; 2333.08088387814; 2308.06565480412; 2282.56034405021; 2256.47287422313; 2229.70428017508; 2202.14968030993; 2173.69998896199; 2144.24368406447; 2113.66758247452; 2081.85585110571; 2048.68725710494; 2014.03141249899; 1977.7449923284; 1939.66849592886; 1899.62342931686; 1857.40930169838; 1812.79975416601; 1765.53721731251; 1715.32525772152; 1661.81700477787; 1604.59703745016; 1543.1534616334; 1476.83692476464; 1404.80240352424; 1325.92091736114; 1238.61667822208; 1140.5102987018; 1027.62017777647; 892.733785613825] kJ/kg  h_w_TLU=[2396.55944251649; 2408.68643343608; 2427.1988031141; 2445.702165897; 2464.18429108356; 2482.62529466839; 2491.82135326629; 2493.6580151792; 2495.49372578218; 2497.32843835745; 2499.16210446923; 2500.99462758899; 2502.83092214066; 2504.6665223621; 2506.50140563013; 2508.335548891; 2510.16892865793; 2519.32352241995; 2537.56068088674; 2555.67742615292; 2573.6403223998; 2591.4109179101; 2608.9455037701; 2626.19492016262; 2643.10444358428; 2659.61377634497; 2675.58278696023; 2696.1846256545; 2716.49989553741; 2736.6235210957; 2756.61216047011; 2776.50561773853; 2796.33378922508; 2816.11979583049; 2835.88181423877; 2855.63430574511; 2875.38889327595; 2895.15500577172; 2914.94035964689; 2934.75132290228; 2954.59319330244; 2974.47041285505; 2994.38673458964; 3014.34535328009; 3034.34900867103; 3054.40006755764; 3074.50058946898; 3094.65237953784; 3114.85703128106; 3135.11596137801; 3155.43043805905; 3175.80160435813] kJ/kg  mu_w_TLU=[6.81365662228272; 7.04953750742707; 7.40970098298307; 7.76991278093907; 8.13017290129507; 8.49048134405107; 8.67065368632907; 8.70668960445667; 8.74272600580827; 8.77876289038387; 8.81480025818347; 8.85083810920707; 8.88687644345467; 8.92291526092627; 8.95895456162187; 8.99499434554147; 9.03103461268507; 9.21124319676307; 9.57169660671907; 9.93219833907507; 10.2927483938311; 10.6533467709871; 11.0139934705431; 11.3746884924991; 11.7354318368551; 12.0962235036111; 12.4570634927671; 12.8179518043231; 13.1788884382791; 13.5398733946351; 13.9009066733911; 14.2619882745471; 14.6231181981031; 14.9842964440591; 15.3455230124151; 15.7067979031711; 16.0681211163271; 16.4294926518831; 16.7909125098391; 17.1523806901951; 17.5138971929511; 17.8754620181071; 18.2370751656631; 18.5987366356191; 18.9604464279751; 19.3222045427311; 19.6840109798871; 20.0458657394431; 20.4077688213991; 20.7697202257551; 21.1317199525111; 21.4937680016671] s*uPa  k_w_TLU=[11.46288215976; 11.941997488935; 12.676358586935; 13.414208884935; 14.155548382935; 14.900377080935; 15.274099879935; 15.348949115735; 15.423833243535; 15.498752263335; 15.573706175135; 15.648694978935; 15.723718674735; 15.798777262535; 15.873870742335; 15.948999114135; 16.024162377935; 16.400502076935; 17.155798374935; 17.914583872935; 18.676858570935; 19.442622468935; 20.211875566935; 20.984617864935; 21.760849362935; 22.540570060935; 23.323779958935; 24.110479056935; 24.900667354935; 25.694344852935; 26.491511550935; 27.292167448935; 28.096312546935; 28.903946844935; 29.715070342935; 30.529683040935; 31.347784938935; 32.169376036935; 32.994456334935; 33.823025832935; 34.655084530935; 35.490632428935; 36.329669526935; 37.172195824935; 38.018211322935; 38.867716020935; 39.720709918935; 40.577193016935; 41.437165314935; 42.300626812935; 43.167577510935; 44.038017408935] mW/m/K  D_w=25 mm^2/s  trace_gas_model=foundation.enum.trace_gas_model.track_fraction  R_g=188.923 J/kg/K  h_g_TLU=[439.555216260064; 444.670268200251; 452.538618847003; 460.487124258496; 468.522588768941; 476.649415958793; 480.74798538725; 481.57054318762; 482.394052398751; 483.218514288831; 484.043930029015; 484.870300696555; 485.697627277859; 486.525910671489; 487.355151691079; 488.185351068185; 489.016509455051; 493.186704139431; 501.599194953048; 510.107689961685; 518.711611080182; 527.410026793075; 536.201764778798; 545.085474203452; 554.059675505208; 563.122805485367; 572.27325096919; 581.509373027928; 590.829525105886; 600.232066705818; 609.715373581392; 619.277845178105; 628.917909922924; 638.634028838794; 648.424697859328; 658.288449140109; 668.223851601449; 678.229510889093; 688.304068901113; 698.44620299875; 708.654624994591; 718.928079991818; 729.265345132425; 739.665228299475; 750.126566808087; 760.648226111439; 771.229098541268; 781.868102096908; 792.564179292476; 803.316296068366; 814.123440770426; 824.984623198037] kJ/kg  mu_g_TLU=[10.8921054191698; 11.2215357085649; 11.7233300740382; 12.2234238147811; 12.7215124453467; 13.2173328890673; 13.4643203184773; 13.5136406274989; 13.562934752385; 13.6122025024997; 13.6614436900741; 13.7106581301692; 13.7598456406398; 13.8090060420983; 13.8581391578796; 13.9072448140062; 13.9563228391538; 14.2012926853717; 14.6890687376044; 15.1738428124161; 15.6554929043332; 16.1339159800463; 16.6090257998657; 17.0807510097148; 17.5490334645512; 18.0138267508952; 18.4750948814453; 18.9328111390399; 19.3869570507278; 19.8375214755778; 20.2844997922255; 20.7278931741254; 21.1677079421287; 21.6039549853963; 22.036649242835; 22.4658092382469; 22.8914566632375; 23.3136160026627; 23.7323141980278; 24.1475803447965; 24.5594454200432; 24.9679420372927; 25.3731042257492; 25.774967231431; 26.1735673380029; 26.5689417053362; 26.9611282240413; 27.350165384404; 27.73609215832; 28.118947892972; 28.4987722151178; 28.8756049449796] s*uPa  k_g_TLU=[10.489430678843; 10.9507672150864; 11.666197960308; 12.392559739764; 13.1299519771612; 13.8778409888416; 14.2554325416312; 14.3312274189707; 14.4071122346908; 14.4830860227061; 14.5591478179508; 14.6352966574703; 14.7115315815553; 14.787851634907; 14.8642558678259; 14.9407433374142; 15.0173131087819; 15.401364480906; 16.1751373988038; 16.9558134611595; 17.7432208682398; 18.5366976599676; 19.3360988502003; 20.1412225692689; 20.9517507672929; 21.7672310558863; 22.5871115634685; 23.4107980865695; 24.2377021890869; 25.0672663781241; 25.8989689893876; 26.732318357514; 27.5668446164644; 28.4020933015927; 29.2376215872816; 30.0729965057542; 30.9077942826816; 31.7416001931033; 32.5740086297993; 33.4046232539953; 34.2330571812868; 35.0589331874899; 35.8818839295189; 36.701552179391; 37.5175910702657; 38.3296643536716; 39.1374466671854; 39.9406238119064; 40.7388930391313; 41.5319633456945; 42.3195557774861; 43.1014037407076] mW/m/K  D_g=16 mm^2/s
  PS-Simulink Converter : nesl_utility/PS-Simulink Converter  PhysicalDomain=network_engine_domain  SubClassName=ps_output  LeftPortType=input  RightPortType=output  PseudoPeriodic=off  Frequencies=[]  VectorFormat=inherit  Unit=W  AffineConversion=off
  PS-Simulink Converter1 : nesl_utility/PS-Simulink Converter  PhysicalDomain=network_engine_domain  SubClassName=ps_output  LeftPortType=input  RightPortType=output  PseudoPeriodic=off  Frequencies=[]  VectorFormat=inherit  Unit=W  AffineConversion=off
  Recirculation Flap : Subsystem  Tag=PublishSubsystem  mask{min_area=1e-8 * cabin_duct_area, max_area=0.9 * cabin_duct_area, port_area=cabin_duct_area, Cd=0.8, tau=1}
      mask prompts: min_area "Min restriction area (m^2)"; max_area "Max restriction area (m^2)"; port_area "Cross-sectional area at ports A, B, and C (m^2)"; Cd "Discharge coefficient"; tau "Opening time constant (s)"
      settings: PortSchema="{\"entries\":[{\"content\":{\"sides\":[{\"content\":{\"connectorIds\":[\"LConn1\"]},\"type\":\"ConnectorPlacement.EquallySpacedRectSide\",\"uuid\":\"955749ca-45ab-4941-92ab-355bdf9f0774\"},{\"content\":{\"connectorIds\":[],\"side\":\"RIGHT\"},\"type\":\"ConnectorPlacement.EquallySpacedRectSide\",\"uuid\":\"c92dcc5f-a0c1-47cb-824d-a6fc82e3fc14\"},{\"content\":{\"connectorIds\":[\"LConn2\"],\"side\":\"TOP\"},\"type\":\"ConnectorPlacement.EquallySpacedRectSide\",\"uuid\":\"48cd19fd-8f40-4cf9-b8e1-bdcb1fb872a4\"},{\"content\":{\"connectorIds\":[\"RConn1\"],\"side\":\"BOTTOM\"},\"type\":\"ConnectorPlacement.EquallySpacedRectSide\",\"uuid\":\"979e7f94-a937-4bda-a98e-05d55fe22e7f\"},{\"content\":{\"connectorIds\":[],\"side\":\"HIDDEN\"},\"type\":\"ConnectorPlacement.EquallySpacedRectSide\",\"uuid\":\"a76ff1f3-0ae3-4e2b-93e3-18e3466b7d92\"}]},\"type\":\"ConnectorPlacement.EquallySpacedConnector\",\"uuid\":\"fbef87af-e9e5-4d13-8a42-ca228c07fa4c\"}],\"packageUris\":[\"http://schema.mathworks.com/mf0/Connector/R2020b\"],\"version\":\"1.0\"}"
  Simulink-PS Converter : nesl_utility/Simulink-PS Converter  PhysicalDomain=network_engine_domain  SubClassName=ps_input  LeftPortType=input  RightPortType=output  PseudoPeriodic=off  Frequencies=[]  NoiseDistribution=none  NoiseParameters=[]  Unit=m^3/s  AffineConversion=off  FilteringAndDerivatives=provide  SimscapeFilterOrder=1  InputFilterTimeConstant=0.001  UdotUserProvided=0
  Simulink-PS Converter1 : nesl_utility/Simulink-PS Converter  PhysicalDomain=network_engine_domain  SubClassName=ps_input  LeftPortType=input  RightPortType=output  PseudoPeriodic=off  Frequencies=[]  NoiseDistribution=none  NoiseParameters=[]  Unit=degC  AffineConversion=on  FilteringAndDerivatives=provide  SimscapeFilterOrder=1  InputFilterTimeConstant=0.001  UdotUserProvided=0
  Simulink-PS Converter2 : nesl_utility/Simulink-PS Converter  PhysicalDomain=network_engine_domain  SubClassName=ps_input  LeftPortType=input  RightPortType=output  PseudoPeriodic=off  Frequencies=[]  NoiseDistribution=none  NoiseParameters=[]  Unit=MPa  AffineConversion=off  FilteringAndDerivatives=provide  SimscapeFilterOrder=1  InputFilterTimeConstant=0.001  UdotUserProvided=0
  Simulink-PS Converter3 : nesl_utility/Simulink-PS Converter  PhysicalDomain=network_engine_domain  SubClassName=ps_input  LeftPortType=input  RightPortType=output  PseudoPeriodic=off  Frequencies=[]  NoiseDistribution=none  NoiseParameters=[]  Unit=1  AffineConversion=off  FilteringAndDerivatives=provide  SimscapeFilterOrder=1  InputFilterTimeConstant=0.001  UdotUserProvided=0
  Simulink-PS Converter4 : nesl_utility/Simulink-PS Converter  PhysicalDomain=network_engine_domain  SubClassName=ps_input  LeftPortType=input  RightPortType=output  PseudoPeriodic=off  Frequencies=[]  NoiseDistribution=none  NoiseParameters=[]  Unit=1  AffineConversion=off  FilteringAndDerivatives=provide  SimscapeFilterOrder=1  InputFilterTimeConstant=0.001  UdotUserProvided=0
  Subtract : Sum  Inputs=+-
  Transfer Fcn : TransferFcn  Denominator=[5 1]
  B : PMIOPort  Side=Left
  A : PMIOPort  Port=2  Side=Right
  tag scope: blower_pwr=global
  wires:
  Max Flow [m^3/s]/1 -> Simulink-PS Converter/1
  Transfer Fcn/1 -> Max Flow [m^3/s]/1
  [T_env] -> Simulink-PS Converter1/1
  [p_env] -> Simulink-PS Converter2/1
  [RH_env] -> Simulink-PS Converter3/1
  [CO2_env] -> Simulink-PS Converter4/1
  PS-Simulink Converter/1 -> Subtract/1
  PS-Simulink Converter1/1 -> Subtract/2
  Subtract/1 -> [blower_pwr]
  [cmd_blower2] -> Transfer Fcn/1
  connections:
  Blower/LConn2 -- Simulink-PS Converter/RConn1
  Moist Air Properties/RConn1 -- Recirculation Flap/LConn2 -- Flow Rate Sensor (MA)/LConn1
  Recirculation Flap/RConn1 -- A/RConn1
  Environment Air/LConn1 -- Recirculation Flap/LConn1
  Simulink-PS Converter1/RConn1 -- Environment Air/RConn1
  Simulink-PS Converter4/RConn1 -- Environment Air/RConn4
  Simulink-PS Converter2/RConn1 -- Environment Air/RConn2
  Simulink-PS Converter3/RConn1 -- Environment Air/RConn3
  Flow Rate Sensor (MA)/RConn1 -- Blower/LConn1
  Flow Rate Sensor (MA)1/RConn1 -- B/RConn1
  Flow Rate Sensor (MA)1/LConn1 -- Blower/RConn1
  PS-Simulink Converter/LConn1 -- Flow Rate Sensor (MA)1/RConn2
  PS-Simulink Converter1/LConn1 -- Flow Rate Sensor (MA)/RConn2
